simulink model "Pure_Pursuit_perhaps"  (R2024b)
settings: Solver=VariableStepAuto  StartTime=0.0  StopTime=10.0  RelTol=1e-3
settings Model: Creator=honor  LastModifiedBy=honor

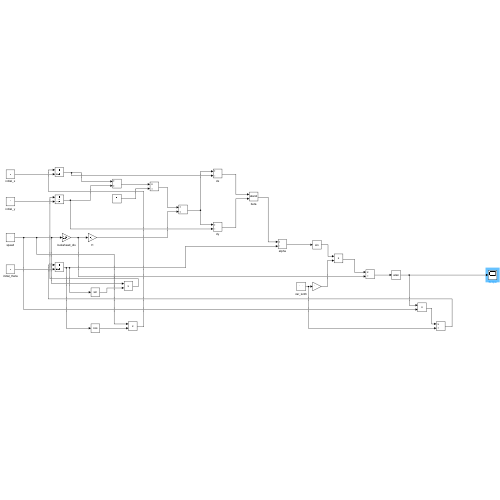
[thumbnail: Simulink's stored preview of the top-level diagram]
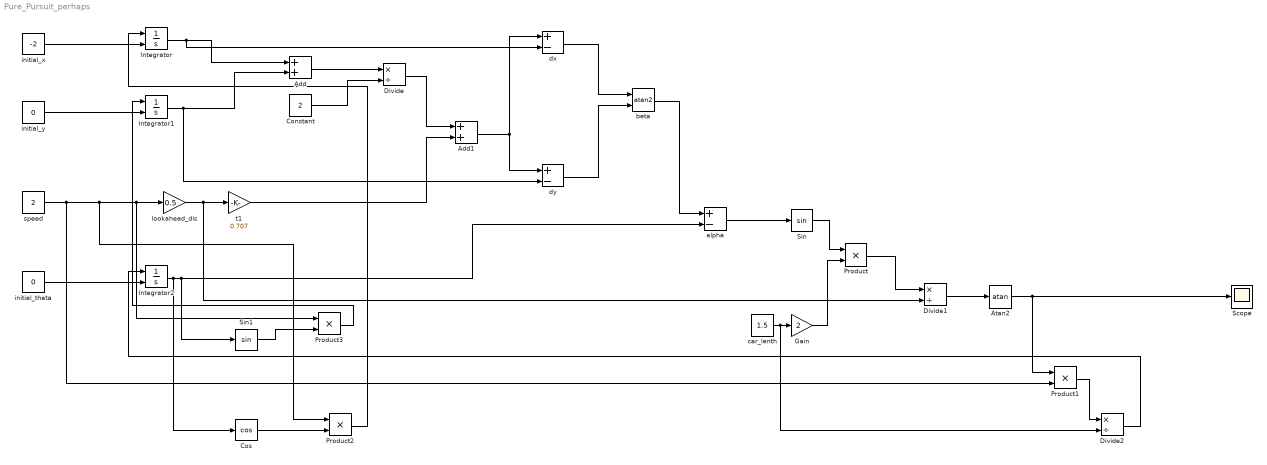
== system Pure_Pursuit_perhaps ==
  Add : Sum
  Add1 : Sum
  Atan2 : Trigonometry  Operator=atan
  Constant : Constant  Value=2
  Cos : Trigonometry  Operator=cos
  Divide : Product  Inputs=*/
  Divide1 : Product  Inputs=*/
  Divide2 : Product  Inputs=*/
  Gain : Gain  Gain=2
  Integrator : Integrator  InitialConditionSource=external
  Integrator1 : Integrator  InitialConditionSource=external
  Integrator2 : Integrator  InitialConditionSource=external
  Product{,1..3} (4 alike) : Product
  Scope : Scope
  Sin : Trigonometry
  Sin1 : Trigonometry
  alpha : Sum  Inputs=+-
  beta : Trigonometry  Operator=atan2
  car_lenth : Constant  Value=1.5
  dx : Sum  Inputs=+-
  dy : Sum  Inputs=+-
  initial_theta : Constant  Value=0
  initial_x : Constant  Value=-2
  initial_y : Constant  Value=0
  lookahead_dis : Gain  Gain=0.5
  speed : Constant  Value=2
  t1 : Gain  Gain=0.707
  wires:
  initial_x/1 -> Integrator/2
  initial_y/1 -> Integrator1/2
  Integrator/1 -> dx/2, Add/1
  Integrator1/1 -> dy/2, Add/2
  initial_theta/1 -> Integrator2/2
  speed/1 -> Product1/2, Product2/1, Product3/1, lookahead_dis/1
  lookahead_dis/1 -> Divide1/2, t1/1
  Add/1 -> Divide/1
  Constant/1 -> Divide/2
  t1/1 -> Add1/2
  Divide/1 -> Add1/1
  Add1/1 -> dy/1, dx/1
  dx/1 -> beta/1
  dy/1 -> beta/2
  Integrator2/1 -> Cos/1, Sin1/1, alpha/2
  beta/1 -> alpha/1
  alpha/1 -> Sin/1
  Sin/1 -> Product/1
  Product/1 -> Divide1/1
  car_lenth/1 -> Divide2/2, Gain/1
  Gain/1 -> Product/2
  Divide1/1 -> Atan2/1
  Atan2/1 -> Product1/1, Scope/1
  Product1/1 -> Divide2/1
  Divide2/1 -> Integrator2/1
  Cos/1 -> Product2/2
  Product2/1 -> Integrator/1
  Sin1/1 -> Product3/2
  Product3/1 -> Integrator1/1
